simulink model "simscapeMultibodyVehicle"  (R2026a)
settings: Solver=FixedStepAuto  StartTime=0  StopTime=60  FixedStep=0.001  MaxStep=0.01  RelTol=1e-2  AbsTol=1e-3
InitFcn:
  | tStop = get_param(bdroot,'StopTime');
StopFcn:
  | active_mode = "AI";
  | if strcmp(get_param([bdroot,'/Vehicle/Driver/PID lateral driver/enable PPU gains'],'Value'), '0')
  |     active_mode = "Static";
  | end
  | fprintf("Active mode: %s\n", active_mode);
  | CTE = get_param([bdroot,'/Dashboard/Display'],'Value');
  | fprintf("Accumulated CTE: %f\n\n", str2double(CTE(3:end-2)));
  | 
  | 
  | % if strcmp(get_param([bdroot,'/Vehicle/Driver/Driver/Lateral Driver'],'ActiveVariant'),'Aurix Red')
  | 
  |     open_system('aurixResetStates','loadonly');
  |     sim('aurixResetStates');
  |     fprintf('AURIX STATES HAVE BEEN RESET\n');
  | 
  | % end
undefined symbols (not defined in the file): ActorRuntime, Defined, Driver, Ego, InitVehicle, Lane, m, Maneuver, n, RRtimeStep, Terrain, User, VehicleData, WheelPoses, X, Y, Z
libraries: nesl_utility x45, sm_lib x42, simulink_extras x7, roadrunnerscenario x6, simscapeMultibodyLibrary x5, etargetslib x4, dspnetwork x4, simulink x1
(part 1 of 4)
settings Model: Creator=The MathWorks, Inc.  LastModifiedBy=chmurski
settings DataIOCC: InspectSignalLogs=on
settings OptimizationCC: SimCompilerOptimization=on
settings SFSimCC: SimCustomHeaderCode="#include \"cast_udp_test.h\""  SFSimEcho=off  DefaultCustomCodeDeterministicFunctions=All  SimHardwareAcceleration=native
settings RTWCC: GenCodeOnly=on  GenerateReport=on
settings SimscapeCC: SimscapeNominalValues="[{\"value\":\"1\",\"unit\":\"A\"},{\"value\":\"1\",\"unit\":\"bar\"},{\"value\":\"1\",\"unit\":\"cm^2\"},{\"value\":\"1\",\"unit\":\"cm^3/s\"},{\"value\":\"1\",\"unit\":\"kJ/kg\"},{\"value\":\"1\",\"unit\":\"kW\"},{\"value\":\"1\",\"unit\":\"l\"},{\"value\":\"1\",\"unit\":\"N\"},{\"value\":\"1\",\"unit\":\"N*m\"},{\"value\":\"1\",\"unit\":\"V\"}]"  SimscapeLogType=none  SimscapeLogDataHistory=5000.0
settings DiagnosticsConfigSet: SimMechanicsConflictingReferenceFrames=none
settings ExplorerConfigSet: SimMechanicsOpenEditorOnUpdate=off  InternalSimMechanicsExplorerSettings="<ExplorerConfiguration><canonicalview>default</canonicalview><AnimationSetting><BasePlaybackSpeed>1.0</BasePlaybackSpeed><PlaybackSpeedFactor>1.0</PlaybackSpeedFactor></AnimationSetting><TilePanel><TileInfo><Tiles Columns=\"2\" Count=\"3\" Rows=\"2\"><Column Weight=\"0.4996\"/><Column Weight=\"0.5004\"/><Row Weight=\"0.4995\"/><Row Weight=\"0.5005\"/><Tile Height=\"1\" Width=\"1\" X=\"0\" Y=\"0\"/><Tile Height=\"1\" Width=\"1\" X=\"0\" Y=\"1\"/><Tile Height=\"2\" Width=\"1\" X=\"1\" Y=\"0\"/></Tiles></TileInfo><SceneInfo><SceneViewer><BGColor><R>0.60000002384185791</R><G>0.60000002384185791</G><B>0.60000002384185791</B></BGColor><Camera><DoPerspective>on</DoPerspective><Position><X>-80.113165366850609</X><Y>-11.1071570914364699</Y><Z>2.41470000000000029</Z></Position><Center><X>-80.9156872814305785</X><Y>-10.5300009199919717</Y><Z>2.26354005033596506</Z></Center><Up><X>-0.122719300806809456</X><Y>0.0882570314021575431</Y><Z>0.988509316909844005</Z></Up><ViewLimDist>1</ViewLimDist><YLim>0.466307658154998583</YLim><XLim>0.581852918582785761</XLim></Camera></SceneViewer><SceneViewer><BGColor><R>0.60000002384185791</R><G>0.60000002384185791</G><B>0.60000002384185791</B></BGColor><Camera><DoPerspective>on</DoPerspective><Position><X>-85.9531653668506124</X><Y>-6.90715709143646617</Y><Z>11.3147000000000002</Z></Position><Center><X>-85.9531653668506124</X><Y>-6.90715709143646617</Y><Z>10.3147000000000002</Z></Center><Up><X>0</X><Y>1</Y><Z>0</Z></Up><ViewLimDist>1</ViewLimDist><YLim>0.466307658154998583</YLim><XLim>0.580568475053905519</XLim></Camera></SceneViewer><SceneViewer><BGColor><R>0.60000002384185791</R><G>0.60000002384185791</G><B>0.60000002384185791</B></BGColor><Camera><DoPerspective>off</DoPerspective><Position><X>51.908161123369787</X><Y>-71.4043721449554027</Y><Z>80.2724563531326112</Z></Position><Center><X>-19.5618792729432052</X><Y>0.0656682513575266857</Y><Z>8.80241595681968114</Z></Center><Up><X>-0.408248290463863073</X><Y>0.408248290463863073</Y><Z>0.816496580927726145</Z></Up><ViewLimDist>1</ViewLimDist><YLim>130.551506244443175</YLim><XLim>80.5591351442734691</XLim></Camera></SceneViewer></SceneInfo></TilePanel><MechEditorPanel><Cameras><Camera><Id>Camera1</Id><Value><Name>FA_FL</Name><NativeCamera><PositionTrackingFeature>Vehicle.Vehicle_Dynamics.Vehicle.Cameras.Frame_FixO_FL.R</PositionTrackingFeature><CenterTrackingFeature>Vehicle.Vehicle_Dynamics.Vehicle.Cameras.Frame_FixO_FL.R</CenterTrackingFeature><UpVectorTrackingFeature>Vehicle.Vehicle_Dynamics.Vehicle.Cameras.Frame_FixO_FL.R</UpVectorTrackingFeature><CenterTrackingOrigin>off</CenterTrackingOrigin><CenterTrackingDirection>+X</CenterTrackingDirection><UpVectorTrackingDirection>+Z</UpVectorTrackingDirection></NativeCamera></Value></Camera><Camera><Id>Camera2</Id><Value><Name>FA_FR</Name><NativeCamera><PositionTrackingFeature>Vehicle.Vehicle_Dynamics.Vehicle.Cameras.Frame_FixO_FR.R</PositionTrackingFeature><CenterTrackingFeature>Vehicle.Vehicle_Dynamics.Vehicle.Cameras.Frame_FixO_FR.R</CenterTrackingFeature><UpVectorTrackingFeature>Vehicle.Vehicle_Dynamics.Vehicle.Cameras.Frame_FixO_FR.R</UpVectorTrackingFeature><CenterTrackingOrigin>off</CenterTrackingOrigin><CenterTrackingDirection>+X</CenterTrackingDirection><UpVectorTrackingDirection>+Z</UpVectorTrackingDirection></NativeCamera></Value></Camera><Camera><Id>Camera3</Id><Value><Name>Top</Name><NativeCamera><PositionTrackingFeature>Vehicle.Vehicle_Dynamics.Vehicle.Cameras.Frame_FixO_Top.R</PositionTrackingFeature><CenterTrackingFeature>Vehicle.Vehicle_Dynamics.Vehicle.Cameras.Frame_FixO_Top.R</CenterTrackingFeature><UpVectorTrackingFeature>Vehicle.Vehicle_Dynamics.Vehicle.Cameras.Frame_FixO_Top.R</UpVectorTrackingFeature><CenterTrackingOrigin>off</CenterTrackingOrigin><CenterTrackingDirection>+X</CenterTrackingDirection><UpVectorTrackingDirection>+Z</UpVectorTrackingDirection></NativeCamera></Value></Camera></Cameras><GfxPanelCameraMap><MapElement CameraMLId=\"Camera2\" GfxPanelIndex=\"0\"/><MapElement CameraMLId=\"Camera3\" GfxPanelIndex=\"1\"/></GfxPanelCameraMap><VideoCreator><PlaybackSpeedRatio>1.0</PlaybackSpeedRatio><FrameRate>30</FrameRate><VideoFormat>Motion JPEG AVI</VideoFormat><FrameSize>auto</FrameSize></VideoCreator></MechEditorPanel></ExplorerConfiguration>"

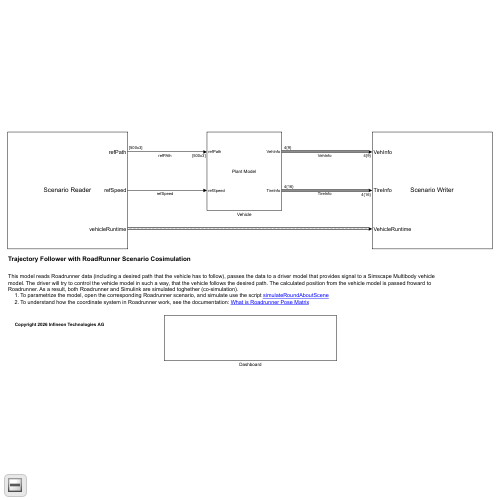
[thumbnail: Simulink's stored preview of the top-level diagram]
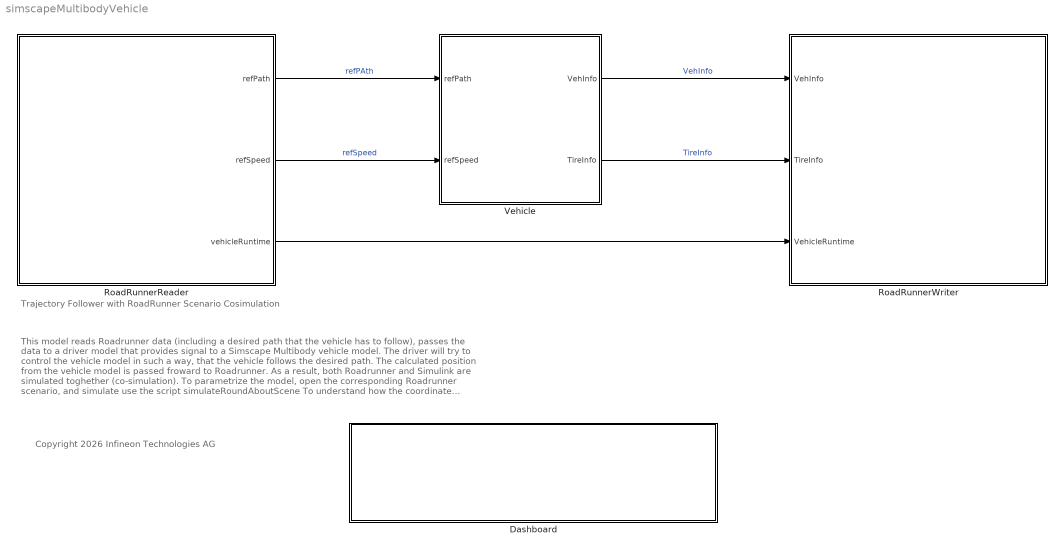
== system simscapeMultibodyVehicle ==
  note: Copyright 2026 Infineon Technologies AG
  note: Trajectory Follower with RoadRunner Scenario Cosimulation
  note: This model reads Roadrunner data (including a desired path that the vehicle has to follow), passes the data to a driver model that provides signal to a Simscape Multibody vehicle model. The driver will try to control the vehicle model in such a way, that the vehicle follows the desired path. The calculated position from the vehicle model is passed froward to Roadrunner. As a result, both Roadrunner and Simulink are simulated toghether (co-simulation).
      | To parametrize the model, open the corresponding Roadrunner scenario, and simulate use the script simulateRoundAboutScene
      | To understand how the coordinate system in Roadrunner work, see the documentation: What is Roadrunner Pose Matrix
  Dashboard : Subsystem
  RoadRunnerReader : Subsystem
      mask Display:
      | % image('ScenarioReader.png')
      | disp('Scenario Reader');
  RoadRunnerWriter : Subsystem
      mask Display:
      | %image('ScenarioWriter.png')
      | disp('Scenario Writer');
  Vehicle : Subsystem
      mask Display:
      | %image('PlantModel.png')
      | disp('Plant Model')
  wires:
  Vehicle/2(TireInfo) -> RoadRunnerWriter/2(TireInfo)  "TireInfo"
  RoadRunnerReader/3(vehicleRuntime) -> RoadRunnerWriter/3(VehicleRuntime)
  RoadRunnerReader/2(refSpeed) -> Vehicle/2(refSpeed)  "refSpeed"
  Vehicle/1(VehInfo) -> RoadRunnerWriter/1(VehInfo)  "VehInfo"
  RoadRunnerReader/1(refPath) -> Vehicle/1(refPath)  "refPAth"

== system simscapeMultibodyVehicle/Dashboard ==
  Dashboard Scope : DashboardScope  FontColor=[0.0, 0.0, 0.0]
  Dashboard Scope1 : DashboardScope  Ymin=0  Ymax=22  ScaleAtStop=off  FontColor=[0.0, 0.0, 0.0]
  Dashboard Scope2 : DashboardScope  Ymin=0  Ymax=15  FontColor=[0.0, 0.0, 0.0]
  Dashboard Scope3 : DashboardScope  Ymin=0  Ymax=15  FontColor=[0.0, 0.0, 0.0]
  Display : DisplayBlock  Transparency=1  GridColor=[0.502, 0.502, 0.502]

== system simscapeMultibodyVehicle/RoadRunnerReader ==
  note: Path Action Reader has a higher time scale since the path does not
      | change during the simulation
  note: Get requested speed from RoadRunner. This has been tested only on the constant speed case for the path following action so far
  All Actor Runtime : roadrunnerscenario/RoadRunner Scenario Reader  Commented=on  TopicCategory=Actor  ActorCategory=All Types  ActionType=Path Following  EventType=User-Defined  TopicType=Actor Pose  VehicleType=Vehicle Specifications  TrafficSignalType=Traffic Signal Specifications  TrafficSignalControllerType=Traffic Signal Controller Specifications  UserDefinedAction=Action1  UserDefinedEvent=Event1  Filter=None  AdditionalRelationship=None  SensorTopic=Target Poses  LaneBoundaryOutputTopic=Ego-Lane  SensorID=1  SampleTime=RRtimeStep
  Constant : Constant  Commented=on  Value=0
  Constant1 : Constant  Value=10
  Cont1 : Subsystem  VariantControl=plantContinuous == 1
      mask Display: disp('Cont')
  MATLAB System : MATLABSystem  System=getPathPoints  timeStep=1  interpNumPoints=500
      mask Type: getPathPoints
  Message Receive : Receive  InputPortMessageModes=m
  Queue : Queue  Commented=on  InputPortMessageModes=m  OutputPortMessageModes=m  OverwriteOldest=on  Capacity=16  QueueType=LIFO
  RoadRunner Scenario : roadrunnerscenario/RoadRunner Scenario  ScenarioFileName=auto  ActorIDLinkedToModel=1  SampleTime=0.02  OpenRoadRunnerAtSimulationStart=on  EnableSimulationLoggingInRoadRunner=off  UserDefinedActions={}  UserDefinedEvents={}  PathPoints=500
  Self Vehicle Runtime : roadrunnerscenario/RoadRunner Scenario Reader  TopicCategory=Actor  ActorCategory=Vehicle  ActionType=Path Following  EventType=User-Defined  TopicType=Actor Specifications  VehicleType=Vehicle Pose  TrafficSignalType=Traffic Signal Specifications  TrafficSignalControllerType=Traffic Signal Controller Specifications  UserDefinedAction=Action1  UserDefinedEvent=Event1  Filter=Self  AdditionalRelationship=None  SensorTopic=Target Poses  LaneBoundaryOutputTopic=Ego-Lane  SensorID=1  SampleTime=RRtimeStep
  Speed Action : roadrunnerscenario/RoadRunner Scenario Reader  Commented=on  TopicCategory=Action  ActorCategory=All Types  ActionType=Speed Change  EventType=User-Defined  TopicType=Actor Specifications  VehicleType=Vehicle Specifications  TrafficSignalType=Traffic Signal Specifications  TrafficSignalControllerType=Traffic Signal Controller Specifications  UserDefinedAction=Action1  UserDefinedEvent=Event1  Filter=Self  AdditionalRelationship=None  SensorTopic=Target Poses  LaneBoundaryOutputTopic=Ego-Lane  SensorID=1  SampleTime=RRtimeStep
  Speed Action Adapter : MATLABSystem  Commented=on  InputPortMessageModes=n,n,n,m,m  System=HelperSpeedActionAdapter
      mask Type: HelperSpeedActionAdapter
  Step Size : Constant  Commented=on  Value=0.01
  To Workspace : ToWorkspace  VariableName=refPath  SaveFormat=Timeseries  SampleTime=-1
  Variant Subsystem : Subsystem  Variant=on  VariantControlMode=label  LabelModeActiveChoice=MoreThan500Points
  refPath : Outport
  refSpeed : Outport  Port=2
  vehicleRuntime : Outport  Port=3
  wires:
  Constant/1 -> Speed Action Adapter/2
  Step Size/1 -> Speed Action Adapter/1
  Variant Subsystem/1(Path) -> MATLAB System/1
  Message Receive/1 -> vehicleRuntime/1
  Speed Action/1 -> Speed Action Adapter/4
  Self Vehicle Runtime/1 -> Message Receive/1
  All Actor Runtime/1 -> Queue/1
  Queue/1 -> Speed Action Adapter/5
  Cont1/1(S) -> refSpeed/1  "refSpeed"
  Variant Subsystem/2(NumPoints) -> MATLAB System/2
  MATLAB System/1 -> refPath/1, To Workspace/1  "refSpeed"
  Constant1/1 -> Cont1/1(In1)

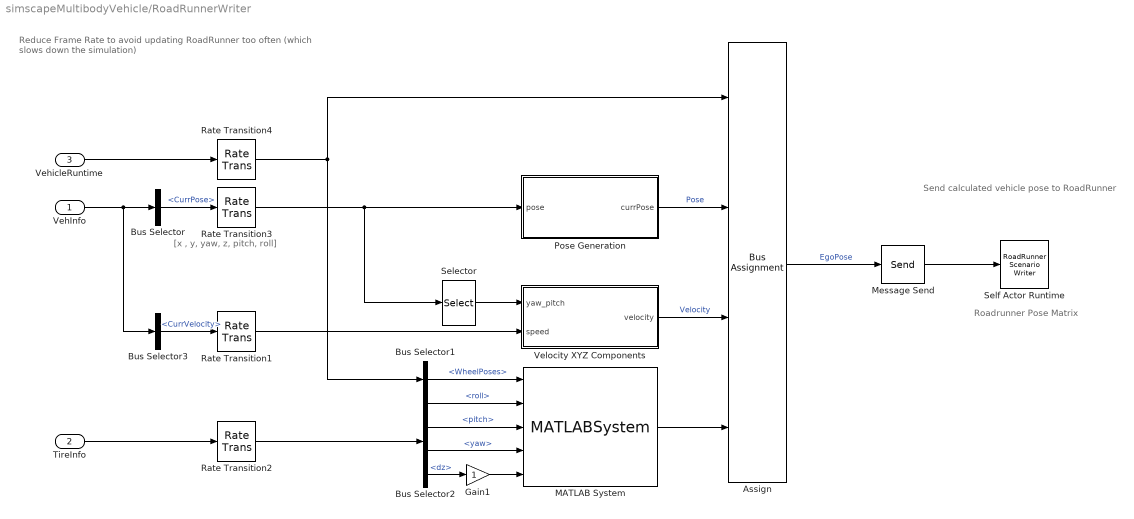
== system simscapeMultibodyVehicle/RoadRunnerWriter ==
  note: [x , y, yaw, z, pitch, roll]
  note: Reduce Frame Rate to avoid updating RoadRunner
      |  too often (which slows down the simulation)
  note: Roadrunner Pose Matrix
  note: Send calculated vehicle pose to RoadRunner
  VehInfo : Inport
  TireInfo : Inport  Port=2
  VehicleRuntime : Inport  Port=3  OutDataTypeStr=Bus: BusVehicleRuntime
  Assign : BusAssignment  AssignedSignals=ActorRuntime.Pose,ActorRuntime.Velocity,WheelPoses
  Bus Selector : BusSelector  OutputSignals=CurrPose
  Bus Selector1 : BusSelector  OutputSignals=WheelPoses
  Bus Selector2 : BusSelector  OutputSignals=roll,pitch,yaw,dz
  Bus Selector3 : BusSelector  OutputSignals=CurrVelocity
  Gain1 : Gain
  MATLAB System : MATLABSystem  System=packWheelPoses  SimulateUsing=Code generation
      mask Type: packWheelPoses
  Message Send : Send  OutputPortMessageModes=m
  Pose Generation : MATLAB Function  TreatAsAtomicUnit=on
  Rate Transition{1..4} (4 alike) : RateTransition  OutPortSampleTime=RRtimeStep
  Selector : Selector  InputPortWidth=6  IndexOptions=Index vector (dialog)  Indices=[3, 5]  OutputSizes=1
  Self Actor Runtime : roadrunnerscenario/RoadRunner Scenario Writer  TopicCategory=Actor  ActorCategory=Vehicle  EventType=Action Complete  UserDefinedEvent=Event1  VehicleType=Vehicle Pose  TopicType=Actor Pose
  Velocity XYZ Components : MATLAB Function  TreatAsAtomicUnit=on
  wires:
  Bus Selector2/3 -> MATLAB System/4  "<yaw>"
  Bus Selector2/2 -> MATLAB System/3  "<pitch>"
  Bus Selector2/1 -> MATLAB System/2  "<roll>"
  Bus Selector2/4 -> Gain1/1  "<dz>"
  Rate Transition3/1 -> Pose Generation/1(pose), Selector/1
  Selector/1 -> Velocity XYZ Components/1(yaw_pitch)
  Bus Selector1/1 -> MATLAB System/1  "<WheelPoses>"
  Gain1/1 -> MATLAB System/5
  Pose Generation/1(currPose) -> Assign/2  "Pose"
  Velocity XYZ Components/1(velocity) -> Assign/3  "Velocity"
  MATLAB System/1 -> Assign/4
  VehicleRuntime/1 -> Rate Transition4/1
  TireInfo/1 -> Rate Transition2/1
  Bus Selector3/1 -> Rate Transition1/1  "<CurrVelocity>"
  VehInfo/1 -> Bus Selector3/1, Bus Selector/1
  Bus Selector/1 -> Rate Transition3/1  "<CurrPose>"
  Rate Transition1/1 -> Velocity XYZ Components/2(speed)
  Message Send/1 -> Self Actor Runtime/1
  Assign/1 -> Message Send/1  "EgoPose"
  Rate Transition2/1 -> Bus Selector2/1
  Rate Transition4/1 -> Bus Selector1/1, Assign/1

== system simscapeMultibodyVehicle/Vehicle ==
  refPath : Inport
  refSpeed : Inport  Port=2
  Driver : Subsystem
      mask Display:
      | %image('DriverModel.png')
      | disp('Driver Model')
  Vehicle Dynamics : Subsystem
      mask Display:
      | % image('PlantModel.png')
      | disp('Vehicle Model')
  VehInfo : Outport
  TireInfo : Outport  Port=2
  wires:
  Driver/2(AccCmd) -> Vehicle Dynamics/2(AccCmd)
  refSpeed/1 -> Driver/3(targetVelocity)
  refPath/1 -> Driver/2(refPath)
  Vehicle Dynamics/2(TireInfo) -> TireInfo/1
  Driver/1(SeerCmd) -> Vehicle Dynamics/1(SteerCmd)
  Vehicle Dynamics/1(VehicleInfo) -> Driver/1(VehicleInfo), VehInfo/1
  Driver/3(DecCmd) -> Vehicle Dynamics/3(DecCmd)

== system simscapeMultibodyVehicle/RoadRunnerReader/Cont1 ==
  In1 : Inport
  Transfer Fcn : TransferFcn  Denominator=[0.01 1]
  S : Outport
  wires:
  Transfer Fcn/1 -> S/1
  In1/1 -> Transfer Fcn/1

== system simscapeMultibodyVehicle/RoadRunnerReader/Variant Subsystem ==
  MoreThan500Points : Subsystem  VariantControl=MoreThan500Points
  Roadrunneer : Subsystem  VariantControl=LessThan500Points
  Path : Outport
  NumPoints : Outport  Port=2

== system simscapeMultibodyVehicle/Vehicle/Driver ==
  VehicleInfo : Inport
  refPath : Inport  Port=2
  targetVelocity : Inport  Port=3
  " Bus Selector" : BusSelector  OutputSignals=gx,aYaw,CurrPose,CurrVelocity
  BreakLoopPose : Subsystem  mask(Body to World){Init=InitVehicle.Vehicle, SpecifyPosTarget=on}
      mask prompts: Init "Initial Values"; SpecifyPosTarget "Specify Position Target"
      mask help: Models the connection between the vehicle body and world. Permits 6 degrees of freedom and sets the initial position, orientation, and speed of the vehicle body.
      mask init:
      | initial_aveh = [Init.yaw Init.pitch Init.roll];
      | rotmat_ypr = sm_vehicle_yawpitchroll_to_rotmat(Init.yaw, Init.pitch, Init.roll);
      | initial_vveh = rotmat_ypr*([Init.vx Init.vy Init.vz])';
      | initial_pxy  = [Init.px Init.py Init.pz];
      mask Help: web('sm_car_doc_body_to_world.html')
  BreakLoopVel : Subsystem  mask(Body to World){Init=InitVehicle.Vehicle, SpecifyPosTarget=on}
      mask prompts: Init "Initial Values"; SpecifyPosTarget "Specify Position Target"
      mask help: Models the connection between the vehicle body and world. Permits 6 degrees of freedom and sets the initial position, orientation, and speed of the vehicle body.
      mask init:
      | initial_aveh = [Init.yaw Init.pitch Init.roll];
      | rotmat_ypr = sm_vehicle_yawpitchroll_to_rotmat(Init.yaw, Init.pitch, Init.roll);
      | initial_vveh = rotmat_ypr*([Init.vx Init.vy Init.vz])';
      mask Help: web('sm_car_doc_body_to_world.html')
  Bus Creator : BusCreator  Inputs=6
  Bus Selector1 : BusSelector  OutputSignals=aSteerWheel,rAccelPedal,rBrakePedal
  Demux : Demux  Outputs=6
  Driver : Subsystem  mask(Driver Behavior){Driver=Driver}
      mask help: Models driver behavior to follow prescribed vehicle trajectory, including path and speed.
  Gain : Gain  Gain=180/pi
  Maneuver : Subsystem  mask(Maneuver Follow Trajectory){Maneuver=Maneuver, popup_window=No}
      mask prompts: popup_window "Check only window of trajectory"
      mask help: Determines target pose to follow prescribed trajectory. Prescribed trajectory is vehicle pose (x, y, theta) and speed along the path to be followed. Optional visual of target pose is also provided.
      mask init:
      | if(strcmpi(get_param(gcb,'popup_window'),'yes'))
      |     set_param([gcb '/window only'],'Value','1');
      | else
      |     set_param([gcb '/window only'],'Value','0');
      | end
      mask TypeOptions popup_window: No | Yes
  PID lateral driver : Subsystem
  Terminator : Terminator
  SeerCmd : Outport  Unit=rad
  AccCmd : Outport  Port=2
  DecCmd : Outport  Port=3
  wires:
  Maneuver/1(vx) -> PID lateral driver/3(CurrVelocity), Driver/1(SpeedIs)
  VehicleInfo/1 -> " Bus Selector"/1
  Demux/6 -> Bus Creator/6  "aRoll"
  Demux/3 -> Bus Creator/3  "aYaw"
  Maneuver/2(Ref) -> PID lateral driver/1(Ref), Driver/2(Ref)
  Driver/1(DrvBus) -> Bus Selector1/1  "Driver"
  Demux/2 -> Bus Creator/2  "y"
  Demux/4 -> Bus Creator/4  "z"
  Bus Creator/1 -> Maneuver/1(VehBus)
  Demux/5 -> Bus Creator/5  "aPitch"
  Maneuver/4(Preview) -> PID lateral driver/2(Preview), Driver/4(Preview)
  Demux/1 -> Bus Creator/1  "x"
  " Bus Selector"/3 -> BreakLoopPose/1(Input)  "<CurrPose>"
  " Bus Selector"/4 -> BreakLoopVel/1(Input)  "<CurrVelocity>"
  Maneuver/3(CurPose) -> Driver/3(CurPose)
  Bus Selector1/2 -> AccCmd/1  "<rAccelPedal>"
  targetVelocity/1 -> Maneuver/4(SpeedRef)
  BreakLoopPose/1(Output) -> Demux/1
  BreakLoopVel/1(Output) -> Maneuver/2(SpeedIs)
  Bus Selector1/3 -> DecCmd/1  "<rBrakePedal>"
  PID lateral driver/1(steering angle AURIX) -> SeerCmd/1
  refPath/1 -> Maneuver/3(Path)
  " Bus Selector"/1 -> PID lateral driver/4(lonAcc)  "<gx>"
  " Bus Selector"/2 -> PID lateral driver/5(yawRate)  "<aYaw>"
  Bus Selector1/1 -> Gain/1  "<aSteerWheel>"
  Gain/1 -> Terminator/1

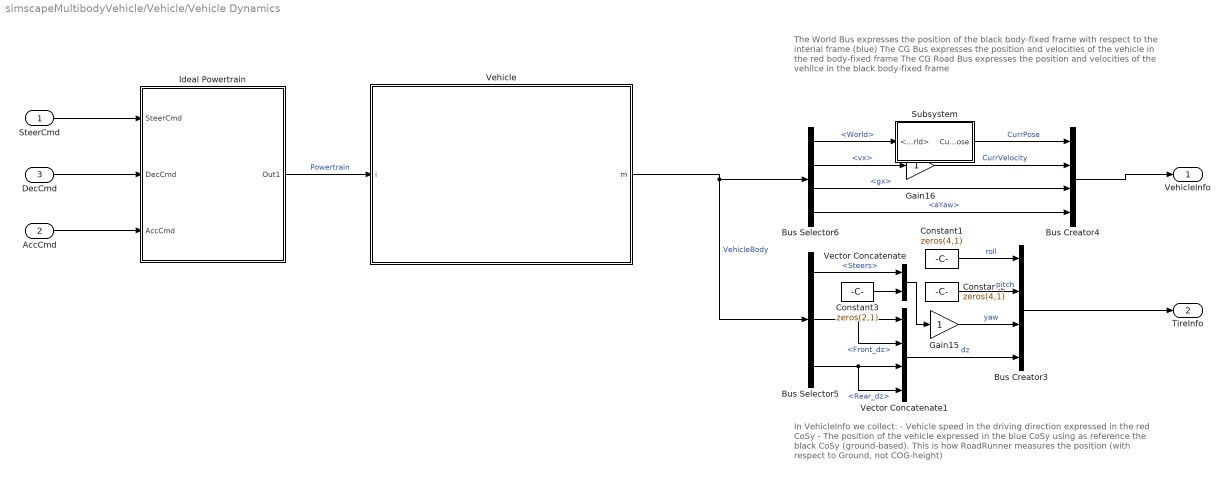
== system simscapeMultibodyVehicle/Vehicle/Vehicle Dynamics ==
  note: The World Bus expresses the position of the black body-fixed
      | frame with respect to the interial frame (blue)
      | The CG Bus expresses the position and velocities of the vehicle
      | in the red body-fixed frame
      | The CG Road Bus expresses the position and velocities of the
      | vehilce in the black body-fixed frame
  note: In VehicleInfo we collect:
      | - Vehicle speed in the driving direction expressed in the red CoSy
      | - The position of the vehicle expressed in the blue CoSy using as
      | reference the black CoSy (ground-based). This is how RoadRunner
      | measures the position (with respect to Ground, not COG-height)
  SteerCmd : Inport
  AccCmd : Inport  Port=2
  DecCmd : Inport  Port=3
  Bus Creator3 : BusCreator  Inputs=4
  Bus Creator4 : BusCreator  Inputs=4
  Bus Selector5 : BusSelector  OutputSignals=Steers,Front_dz,Rear_dz
  Bus Selector6 : BusSelector  OutputSignals=World,CG.vx,CG.gx,World.aYaw
  Constant1 : Constant  Value=zeros(4,1)
  Constant2 : Constant  Value=zeros(4,1)
  Constant3 : Constant  Value=zeros(2,1)
  Gain15 : Gain
  Gain16 : Gain
  Ideal Powertrain : Subsystem
  Subsystem : Subsystem
  Vector Concatenate : Concatenate
  Vector Concatenate1 : Concatenate  NumInputs=4
  Vehicle : Subsystem  mask(Vehicle and Scene){vehdata=VehicleData, initveh=InitVehicle, terrain=Terrain}
      mask prompts: vehdata "Vehicle Data (structure)"; initveh "Initial Position, Velocity (structure)"; terrain "Terrain Data"
      mask help: Models a vehicle with a configurable scene. Vehicle parameters are defined within a single data structure. A separate data structure defines the initial position, orientation, and speed of the vehicle and the wheels.
      mask Display: image('TopLevel.png')
  VehicleInfo : Outport
  TireInfo : Outport  Port=2
  wires:
  Vehicle/1(m) -> Bus Selector5/1, Bus Selector6/1  "VehicleBody"
  Constant3/1 -> Vector Concatenate/2
  Bus Selector5/1 -> Vector Concatenate/1  "<Steers>"
  Bus Creator3/1 -> TireInfo/1
  Gain16/1 -> Bus Creator4/2  "CurrVelocity"
  Bus Creator4/1 -> VehicleInfo/1
  Constant1/1 -> Bus Creator3/1  "roll"
  Subsystem/1(CurrPose) -> Bus Creator4/1  "CurrPose"
  Bus Selector6/1 -> Subsystem/1(<World>)  "<World>"
  Constant2/1 -> Bus Creator3/2  "pitch"
  Bus Selector5/2 -> Vector Concatenate1/2, Vector Concatenate1/1  "<Front_dz>"
  Vector Concatenate/1 -> Gain15/1
  Gain15/1 -> Bus Creator3/3  "yaw"
  Bus Selector6/2 -> Gain16/1  "<vx>"
  Vector Concatenate1/1 -> Bus Creator3/4  "dz"
  Bus Selector5/3 -> Vector Concatenate1/4, Vector Concatenate1/3  "<Rear_dz>"
  Ideal Powertrain/1(Out1) -> Vehicle/1(i)  "Powertrain"
  SteerCmd/1 -> Ideal Powertrain/1(SteerCmd)
  DecCmd/1 -> Ideal Powertrain/2(DecCmd)
  AccCmd/1 -> Ideal Powertrain/3(AccCmd)
  Bus Selector6/3 -> Bus Creator4/3  "<gx>"
  Bus Selector6/4 -> Bus Creator4/4  "<aYaw>"

== system simscapeMultibodyVehicle/RoadRunnerReader/Variant Subsystem/MoreThan500Points ==
  Bus Selector2 : BusSelector  OutputSignals=Path,NumPoints
  MATLAB System1 : MATLABSystem  System=HelperPathActionReader  sampleTime=-1
      mask Type: HelperPathActionReader
  Path : Outport
  NumPoints : Outport  Port=2
  wires:
  Bus Selector2/1 -> Path/1  "<Path>"
  Bus Selector2/2 -> NumPoints/1  "<NumPoints>"
  MATLAB System1/1 -> Bus Selector2/1

== system simscapeMultibodyVehicle/RoadRunnerReader/Variant Subsystem/Roadrunneer ==
  Bus Selector2 : BusSelector  OutputSignals=Path,NumPoints
  Message Receive1 : Receive  InputPortMessageModes=m
  PathActionReader : roadrunnerscenario/RoadRunner Scenario Reader  TopicCategory=Action  ActorCategory=Vehicle  ActionType=Path Following  EventType=User-Defined  TopicType=Actor Specifications  VehicleType=Vehicle Pose  UserDefinedAction=Action1  UserDefinedEvent=Event1  Filter=Self  SensorTopic=Target Poses  LaneBoundaryOutputTopic=Ego-Lane  SensorID=1  SampleTime=RRtimeStep*10
  Path : Outport
  NumPoints : Outport  Port=2
  wires:
  Message Receive1/1 -> Bus Selector2/1
  PathActionReader/1 -> Message Receive1/1
  Bus Selector2/1 -> Path/1  "<Path>"
  Bus Selector2/2 -> NumPoints/1  "<NumPoints>"

== system simscapeMultibodyVehicle/Vehicle/Driver/BreakLoopPose ==
  Input : Inport
  Demux : Demux  Outputs=6
  Mux : Mux  Inputs=6
  Transfer Fcn : TransferFcn  Denominator=[1 1]
  Transfer Fcn (with initial outputs) : simulink_extras/Additional Linear/Transfer Fcn (with initial outputs)  N=[1]  D="[0.01  1]"  Y0=initial_pxy(1)  U0=initial_pxy(1)
  Transfer Fcn (with initial outputs)1 : simulink_extras/Additional Linear/Transfer Fcn (with initial outputs)  N=[1]  D="[0.01  1]"  Y0=initial_pxy(2)  U0=initial_pxy(2)
  Transfer Fcn (with initial outputs)2 : simulink_extras/Additional Linear/Transfer Fcn (with initial outputs)  N=[1]  D="[0.01  1]"  Y0=initial_pxy(3)  U0=initial_pxy(3)
  Transfer Fcn (with initial outputs)3 : simulink_extras/Additional Linear/Transfer Fcn (with initial outputs)  N=[1]  D="[0.01  1]"  Y0=initial_aveh(1)  U0=initial_aveh(1)
  Transfer Fcn (with initial outputs)4 : simulink_extras/Additional Linear/Transfer Fcn (with initial outputs)  N=[1]  D="[0.01  1]"  Y0=initial_aveh(2)  U0=initial_aveh(2)
  Transfer Fcn (with initial outputs)5 : simulink_extras/Additional Linear/Transfer Fcn (with initial outputs)  N=[1]  D="[0.01  1]"  Y0=initial_aveh(3)  U0=initial_aveh(3)
  Output : Outport
  wires:
  Mux/1 -> Output/1  "CurrPose"
  Input/1 -> Demux/1
  Transfer Fcn (with initial outputs)2/1 -> Mux/4  "z"
  Transfer Fcn (with initial outputs)/1 -> Mux/1  "x"
  Demux/4 -> Transfer Fcn (with initial outputs)2/1
  Transfer Fcn (with initial outputs)4/1 -> Mux/5  "aPitch"
  Demux/6 -> Transfer Fcn (with initial outputs)5/1
  Transfer Fcn (with initial outputs)3/1 -> Mux/3  "aYaw"
  Transfer Fcn (with initial outputs)5/1 -> Mux/6  "aRoll"
  Demux/5 -> Transfer Fcn (with initial outputs)4/1
  Transfer Fcn (with initial outputs)1/1 -> Mux/2  "y"
  Demux/2 -> Transfer Fcn (with initial outputs)1/1
  Demux/1 -> Transfer Fcn (with initial outputs)/1
  Demux/3 -> Transfer Fcn (with initial outputs)3/1

== system simscapeMultibodyVehicle/Vehicle/Driver/BreakLoopVel ==
  Input : Inport
  Transfer Fcn (with initial outputs) : simulink_extras/Additional Linear/Transfer Fcn (with initial outputs)  N=[1]  D="[0.01  1]"  Y0=initial_vveh(1)  U0=initial_vveh(1)
  Output : Outport
  wires:
  Transfer Fcn (with initial outputs)/1 -> Output/1
  Input/1 -> Transfer Fcn (with initial outputs)/1

== system simscapeMultibodyVehicle/Vehicle/Driver/Driver ==
  SpeedIs : Inport
  Ref : Inport  Port=2
  CurPose : Inport  Port=3
  Preview : Inport  Port=4
  Bus Creator5 : BusCreator  Inputs=4
  Bus Selector1 : BusSelector  OutputSignals=vTarget
  Bus Selector2 : BusSelector  OutputSignals=dist
  Constant9 : Constant  Value=0
  Cur Pose : Subsystem
  Filter Steer Cmd : TransferFcn  Denominator=[1/Driver.Lateral.fSteerCutoff.Value 1]
  Fwd Rev : Subsystem
  Lateral Driver : Subsystem  Variant=on  VariantControlMode=label  VariantControl=Choice  LabelModeActiveChoice=Stanley  mask{Lateral=Driver.Lateral}
      mask prompts: Lateral "Lateral Driver Parameters (structure)"
  Longitudinal Driver : Subsystem  mask(Longitudinal Driver (Velocity-tracking Controller)){SPEED_LOOKAHEAD_TIME=Driver.Long.FFLookahead.Value, C_ROLLING_RESISTANCE_COEFF=Driver.Long.NRollingResistance.Value, ROAD_FRICTION_COEFF=Driver.Long.NRoadFriction.Value, mVehicle=Driver.Long.mVehicle.Value, gGravity=Driver.Long.gGravity.Value, FTractive=Driver.Long.FTractive.Value, KP_SPEED=Driver.Long.Kp.Value, KI_SPEED=Driver.Long.Ki.Value, MAX_ACCEL_MPS2=Driver.Long.gMaxAccel.Value, MAX_DECEL_MPS2=Driver.Long.gMaxDecel.Value, Cdrag=0.23, rho_air=1.255, ARef=2.3}
      mask prompts: SPEED_LOOKAHEAD_TIME "Lookahead time (s)"; C_ROLLING_RESISTANCE_COEFF "Rolling resistance coefficient"; ROAD_FRICTION_COEFF "Road friction coefficient"; mVehicle "Total Vehicle mass (kg)"; gGravity "Gravity (m/s)"; FTractive "Tractive Force (N)"; KP_SPEED "Proportional gain, Kp"; KI_SPEED "Integral gain, Ki"; MAX_ACCEL_MPS2 "Max acceleration (m/s^2, positive number))"; MAX_DECEL_MPS2 "Max deceleration (m/s^2, must be negative)"; Cdrag "Drag coefficient"; rho_air "Density of air (kg/m^3)"; ARef "Frontal Area (m^2)"
      mask help: Implements a PI controller with feedforward for velocity tracking.
      mask DialogControl cont_feedforward Prompt: Feed-Forward Controller parameters
      mask DialogControl cont_feedback Prompt: Feedback Controller parameters
      mask DialogControl cont_drag Prompt: Drag
  Ref Pose and Distance : Subsystem
  Transfer Fcn : TransferFcn  Denominator=[1/(Driver.Long.fAccelCutoff.Value) 1]
  Transfer Fcn1 : TransferFcn  Denominator=[1/(Driver.Long.fBrakeCutoff.Value) 1]
  DrvBus : Outport  VectorParamsAs1DForOutWhenUnconnected=off
  wires:
  Bus Selector2/1 -> Longitudinal Driver/4(Distance)  "<dist>"
  Fwd Rev/2(vxFwRv) -> Longitudinal Driver/3(vx)
  Bus Selector1/1 -> Fwd Rev/2(vT)  "<vTarget>"
  Ref Pose and Distance/2(Dist) -> Lateral Driver/2(Distance)
  Preview/1 -> Longitudinal Driver/1(Preview)
  Lateral Driver/1(steeringAngle) -> Filter Steer Cmd/1
  Fwd Rev/1(dir) -> Lateral Driver/5(Direction), Longitudinal Driver/2(dir)
  SpeedIs/1 -> Fwd Rev/1(vx), Lateral Driver/4(v_x)
  Cur Pose/1(CurPose) -> Lateral Driver/3(currentPose)
  CurPose/1 -> Cur Pose/1(Cur)
  Constant9/1 -> Longitudinal Driver/5(current_slope_rad)
  Bus Creator5/1 -> DrvBus/1  "DrvBus"
  Longitudinal Driver/1(AccelCmd) -> Transfer Fcn/1
  Longitudinal Driver/2(DecelCmd) -> Transfer Fcn1/1
  Transfer Fcn1/1 -> Bus Creator5/4  "rBrakePedal"
  Transfer Fcn/1 -> Bus Creator5/3  "rAccelPedal"
  Ref/1 -> Bus Creator5/1, Bus Selector1/1, Bus Selector2/1, Ref Pose and Distance/1(Ref)
  Ref Pose and Distance/1(RefPose) -> Lateral Driver/1(referencePose)
  Filter Steer Cmd/1 -> Bus Creator5/2  "aSteerWheel"

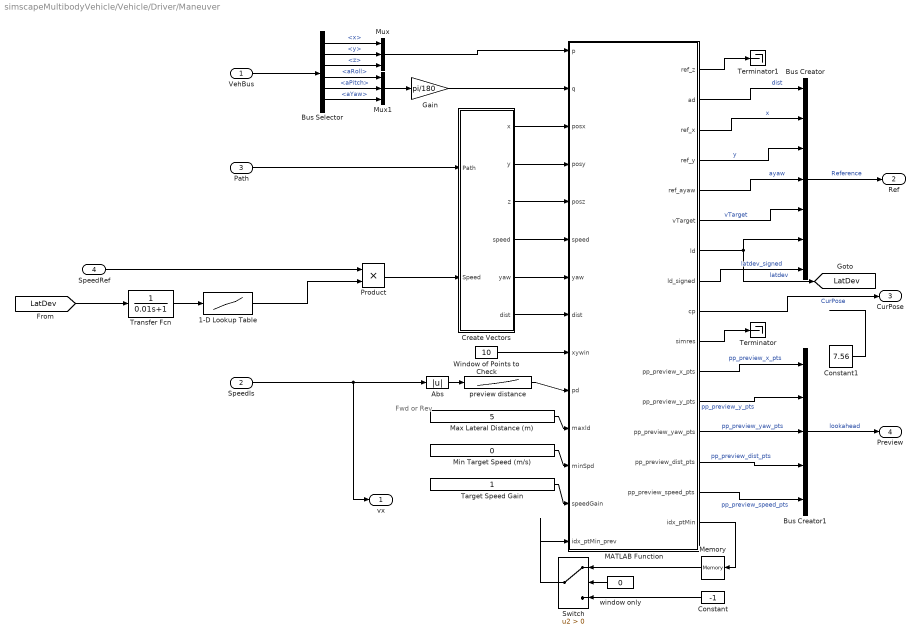
== system simscapeMultibodyVehicle/Vehicle/Driver/Maneuver ==
  note: Fwd or
      | Rev
  VehBus : Inport
  SpeedIs : Inport  Port=2
  Path : Inport  Port=3
  SpeedRef : Inport  Port=4
  1-D Lookup Table : Lookup_n-D  NumberOfTableDimensions=1  BreakpointsForDimension1=[0,0.5,1,2]  Table=[1, 0.8, 0.5, 0.1]  InternalRulePriority=Speed  RndMeth=Simplest
  Abs : Abs  ZeroCross=off  SaturateOnIntegerOverflow=off
  Bus Creator : BusCreator  Inputs=7
  Bus Creator1 : BusCreator  Inputs=5
  Bus Selector : BusSelector  OutputSignals=x,y,z,aRoll,aPitch,aYaw
  Constant : Constant  Value=-1
  Constant1 : Constant  Value=7.56  OutDataTypeStr=Inherit: Inherit via back propagation  SampleTime=-1
  Create Vectors : MATLAB Function  TreatAsAtomicUnit=on
  Gain : Gain  Gain=pi/180
  MATLAB Function : MATLAB Function  SystemSampleTime=0.1  mask{nPreviewPoints=50}
      mask prompts: nPreviewPoints "Number of Preview Points"
  Max Lateral Distance (m) : Constant  Value=5
  Memory : Memory  InitialCondition=-1
  Min Target Speed (m/s) : Constant  Value=0
  Mux : Mux  Inputs=3
  Mux1 : Mux  Inputs=3
  Product : Product
  Switch : Switch  Criteria=u2 > Threshold  SaturateOnIntegerOverflow=off  InputSameDT=off
  Target Speed Gain : Constant
  Terminator : Terminator
  Terminator1 : Terminator
  Transfer Fcn : TransferFcn  Denominator=[0.01 1]
  Window of Points to Check : Constant  Value=10
  preview distance : Lookup_n-D  NumberOfTableDimensions=1  BreakpointsForDimension1=Maneuver.xPreview.v.Value  Table=Maneuver.xPreview.x.Value  InternalRulePriority=Speed  RndMeth=Simplest
  window only : Constant  Value=0
  vx : Outport  VectorParamsAs1DForOutWhenUnconnected=off
  Ref : Outport  Port=2  VectorParamsAs1DForOutWhenUnconnected=off
  CurPose : Outport  Port=3  VectorParamsAs1DForOutWhenUnconnected=off
  Preview : Outport  Port=4  VectorParamsAs1DForOutWhenUnconnected=off
  tag scope: LatDev=global
  wires:
  MATLAB Function/15(pp_preview_speed_pts) -> Bus Creator1/5  "pp_preview_speed_pts"
  SpeedIs/1 -> Abs/1, vx/1
  VehBus/1 -> Bus Selector/1
  Bus Creator1/1 -> Preview/1  "lookahead"
  MATLAB Function/14(pp_preview_dist_pts) -> Bus Creator1/4  "pp_preview_dist_pts"
  MATLAB Function/13(pp_preview_yaw_pts) -> Bus Creator1/3  "pp_preview_yaw_pts"
  MATLAB Function/12(pp_preview_y_pts) -> Bus Creator1/2  "pp_preview_y_pts"
  MATLAB Function/11(pp_preview_x_pts) -> Bus Creator1/1  "pp_preview_x_pts"
  MATLAB Function/7(ld) -> [LatDev], Bus Creator/6  "latdev"
  Min Target Speed (m/s)/1 -> MATLAB Function/12(minSpd)
  Target Speed Gain/1 -> MATLAB Function/13(speedGain)
  Max Lateral Distance (m)/1 -> MATLAB Function/11(maxld)
  Bus Selector/1 -> Mux/1  "<x>"
  Mux1/1 -> Gain/1
  Mux/1 -> MATLAB Function/1(p)
  MATLAB Function/3(ref_x) -> Bus Creator/2  "x"
  MATLAB Function/9(cp) -> CurPose/1  "CurPose"
  preview distance/1 -> MATLAB Function/10(pd)
  MATLAB Function/4(ref_y) -> Bus Creator/3  "y"
  MATLAB Function/5(ref_ayaw) -> Bus Creator/4  "ayaw"
  MATLAB Function/2(ad) -> Bus Creator/1  "dist"
  Bus Creator/1 -> Ref/1  "Reference"
  MATLAB Function/6(vTarget) -> Bus Creator/5  "vTarget"
  MATLAB Function/10(simres) -> Terminator/1
  Window of Points to Check/1 -> MATLAB Function/9(xywin)
  MATLAB Function/16(idx_ptMin) -> Memory/1
  Switch/1 -> MATLAB Function/14(idx_ptMin_prev)
  Constant/1 -> Switch/3
  window only/1 -> Switch/2
  Memory/1 -> Switch/1
  Abs/1 -> preview distance/1
  Bus Selector/6 -> Mux1/3  "<aYaw>"
  Bus Selector/5 -> Mux1/2  "<aPitch>"
  Bus Selector/4 -> Mux1/1  "<aRoll>"
  Bus Selector/2 -> Mux/2  "<y>"
  Bus Selector/3 -> Mux/3  "<z>"
  Gain/1 -> MATLAB Function/2(q)
  Path/1 -> Create Vectors/1(Path)
  Create Vectors/6(dist) -> MATLAB Function/8(dist)
  Create Vectors/5(yaw) -> MATLAB Function/7(yaw)
  Create Vectors/4(speed) -> MATLAB Function/6(speed)
  Create Vectors/3(z) -> MATLAB Function/5(posz)
  Create Vectors/2(y) -> MATLAB Function/4(posy)
  Create Vectors/1(x) -> MATLAB Function/3(posx)
  MATLAB Function/1(ref_z) -> Terminator1/1
  [LatDev] -> Transfer Fcn/1
  Transfer Fcn/1 -> 1-D Lookup Table/1
  SpeedRef/1 -> Product/1
  Product/1 -> Create Vectors/2(Speed)
  1-D Lookup Table/1 -> Product/2
  MATLAB Function/8(ld_signed) -> Bus Creator/7  "latdev_signed"
  Constant1/1 -> ?

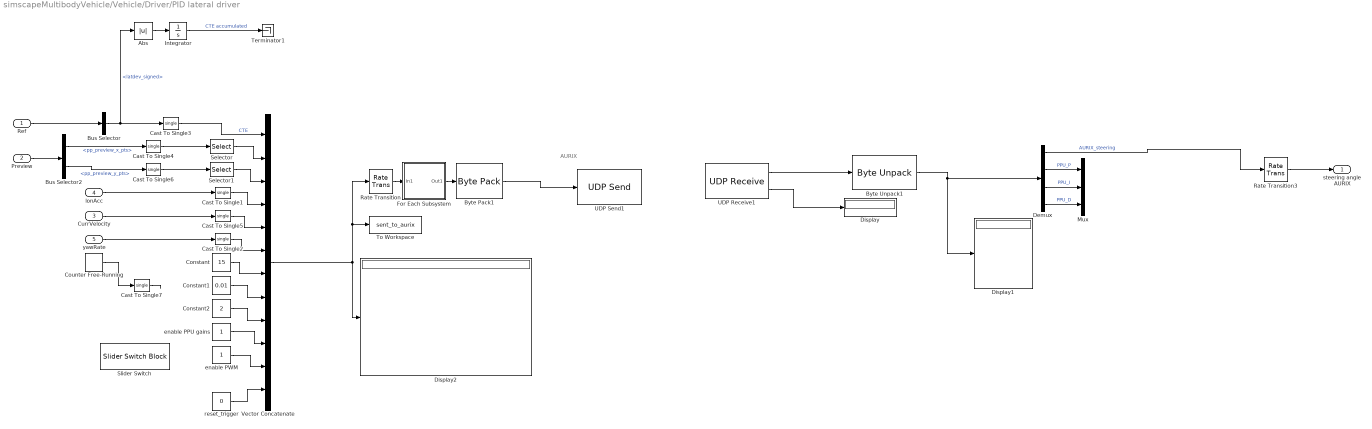
== system simscapeMultibodyVehicle/Vehicle/Driver/PID lateral driver ==
  note: AURIX
  Ref : Inport
  Preview : Inport  Port=2
  CurrVelocity : Inport  Port=3
  lonAcc : Inport  Port=4
  yawRate : Inport  Port=5
  Abs : Abs  SaturateOnIntegerOverflow=off
  Bus Selector : BusSelector  OutputSignals=latdev_signed
  Bus Selector2 : BusSelector  OutputSignals=pp_preview_x_pts,pp_preview_y_pts
  Byte Pack1 : etargetslib/Byte Pack  datatypes={'uint32'}  byteAlign=1
  Byte Unpack1 : etargetslib/Byte Unpack  dimensions={[4]}  datatypes={'single'}  byteAlign=1
      settings: LibrarySourceBlock=embeddedtargetslib/Host Communication/Byte Unpack
  Cast To Single{1..7} (7 alike) : DataTypeConversion  OutDataTypeStr=single  SaturateOnIntegerOverflow=off  RndMeth=Floor
  Constant : Constant  Value=15  OutDataTypeStr=single
  Constant1 : Constant  Value=0.01  OutDataTypeStr=single
  Constant2 : Constant  Value=2  OutDataTypeStr=single
  Counter Free-Running : simulink/Sources/Counter Free-Running  NumBits=32  tsamp=0.01
  Demux : Demux
  Display : Display
  Display1 : Display
  Display2 : Display
  For Each Subsystem : Subsystem  TreatAsAtomicUnit=on
  Integrator : Integrator
  Mux : Mux  Inputs=3
  Rate Transition : RateTransition  OutPortSampleTime=0.01
  Rate Transition3 : RateTransition
  Selector : Selector  NumberOfDimensions=2  InputPortWidth=50  IndexOptions=Index vector (dialog),Index vector (dialog)  Indices=1,[1:10:50]  OutputSizes=1,1
  Selector1 : Selector  NumberOfDimensions=2  InputPortWidth=50  IndexOptions=Index vector (dialog),Index vector (dialog)  Indices=1,[1:10:50]  OutputSizes=1,1
  Slider Switch : SliderSwitchBlock
  Terminator1 : Terminator
  To Workspace : ToWorkspace  VariableName=sent_to_aurix  SaveFormat=Timeseries  SampleTime=-1
  UDP Receive1 : dspnetwork/UDP Receive  localURL='0.0.0.0'  localPort=55555  remoteURL='192.168.178.5'  remotePort=-1  recvBufferSize=4*4  dims=4*4  signalDatatype=uint8  isComplex=off  isVarSize=off  showBlockingTime=on  blockingTime=0  sampletime=0.01  blockPlatform=HOST
      settings: LibrarySourceBlock=embeddedtargetslib/Host Communication/UDP Receive
  UDP Send1 : dspnetwork/UDP Send  remoteURL='192.168.178.5'  remotePort=2300  localURL='0.0.0.0'  localPortSource=Specify via dialog  localPort=55555  sendBufferSize=20*4  sampletime=-1  blockPlatform=HOST  separateLengthPort=0
      settings: LibrarySourceBlock=embeddedtargetslib/Host Communication/UDP Send
  Vector Concatenate : Concatenate  NumInputs=12
  enable PPU gains : Constant  OutDataTypeStr=single
  enable PWM : Constant  OutDataTypeStr=single
  reset_trigger : Constant  Value=0  OutDataTypeStr=single
  steering angle AURIX : Outport
  wires:
  Ref/1 -> Bus Selector/1
  Preview/1 -> Bus Selector2/1
  UDP Receive1/1 -> Byte Unpack1/1
  Vector Concatenate/1 -> Rate Transition/1, To Workspace/1, Display2/1
  Byte Pack1/1 -> UDP Send1/1
  For Each Subsystem/1(Out1) -> Byte Pack1/1
  Bus Selector2/1 -> Cast To Single4/1  "<pp_preview_x_pts>"
  Bus Selector2/2 -> Cast To Single6/1  "<pp_preview_y_pts>"
  lonAcc/1 -> Cast To Single1/1
  CurrVelocity/1 -> Cast To Single5/1
  yawRate/1 -> Cast To Single2/1
  Cast To Single5/1 -> Vector Concatenate/5
  Cast To Single1/1 -> Vector Concatenate/4
  Cast To Single2/1 -> Vector Concatenate/6
  Cast To Single3/1 -> Vector Concatenate/1  "CTE"
  Selector1/1 -> Vector Concatenate/3
  Selector/1 -> Vector Concatenate/2
  Cast To Single4/1 -> Selector/1
  Cast To Single6/1 -> Selector1/1
  UDP Receive1/2 -> Display/1
  Bus Selector/1 -> Abs/1, Cast To Single3/1  "<latdev_signed>"
  Rate Transition/1 -> For Each Subsystem/1(In1)
  Byte Unpack1/1 -> Demux/1, Display1/1
  Counter Free-Running/1 -> Cast To Single7/1
  Cast To Single7/1 -> ?
  Demux/1 -> Rate Transition3/1  "AURIX_steering"
  Constant2/1 -> Vector Concatenate/9
  Constant1/1 -> Vector Concatenate/8
  Constant/1 -> Vector Concatenate/7
  enable PPU gains/1 -> Vector Concatenate/10
  Integrator/1 -> Terminator1/1  "CTE accumulated"
  Abs/1 -> Integrator/1
  Rate Transition3/1 -> steering angle AURIX/1
  enable PWM/1 -> Vector Concatenate/11
  reset_trigger/1 -> Vector Concatenate/12
  Demux/2 -> Mux/1  "PPU_P"
  Demux/3 -> Mux/2  "PPU_I"
  Demux/4 -> Mux/3  "PPU_D"

== system simscapeMultibodyVehicle/Vehicle/Vehicle Dynamics/Ideal Powertrain ==
  SteerCmd : Inport
  DecCmd : Inport  Port=2
  AccCmd : Inport  Port=3
  Bus Creator : BusCreator  Inputs=5
  Gain{,1..3} (4 alike) : Gain
  Gain5 : Gain  Gain=-1
  SteeringWheelRatio : Gain  Gain=VehicleData.SuspF.SteerRatio
  Switch : Switch  Criteria=u2 > Threshold  Threshold=0.1  SaturateOnIntegerOverflow=off  InputSameDT=off
  TorqueScaler : Gain  Gain=1.3*VehicleData.Body.Mass/4*0.35
  deg2rad : Gain  Gain=pi/180
  Out1 : Outport
  wires:
  Gain2/1 -> Bus Creator/4  "trqRR"
  SteerCmd/1 -> SteeringWheelRatio/1
  deg2rad/1 -> Bus Creator/1  "sWhl"
  DecCmd/1 -> Gain5/1, Switch/2
  Gain/1 -> Bus Creator/2  "trqFR"
  TorqueScaler/1 -> Gain/1, Gain1/1, Gain3/1, Gain2/1
  Switch/1 -> TorqueScaler/1
  Gain3/1 -> Bus Creator/5  "trqRL"
  Gain5/1 -> Switch/1
  SteeringWheelRatio/1 -> deg2rad/1  "sWhl"
  Gain1/1 -> Bus Creator/3  "trqFL"
  Bus Creator/1 -> Out1/1
  AccCmd/1 -> Switch/3

== system simscapeMultibodyVehicle/Vehicle/Vehicle Dynamics/Subsystem ==
  <World> : Inport
  Bus Selector7 : BusSelector  OutputSignals=x,y,aYaw,z,aPitch,aRoll
  Gain1 : Gain  Gain=180/pi
  Gain18 : Gain  Gain=180/pi
  Gain2 : Gain  Gain=180/pi
  Mux1 : Mux  Inputs=6
  CurrPose : Outport
  wires:
  Bus Selector7/5 -> Gain1/1  "<aPitch>"
  Bus Selector7/2 -> Mux1/2  "<y>"
  Gain18/1 -> Mux1/3  "yaw_deg"
  <World>/1 -> Bus Selector7/1
  Bus Selector7/1 -> Mux1/1  "<x>"
  Bus Selector7/3 -> Gain18/1  "<aYaw>"
  Mux1/1 -> CurrPose/1  "CurrPose"
  Bus Selector7/4 -> Mux1/4  "<z>"
  Bus Selector7/6 -> Gain2/1  "<aRoll>"
  Gain1/1 -> Mux1/5  "pitch_deg"
  Gain2/1 -> Mux1/6  "roll_deg"
